simulink model "NMC_batt_model_80_1dot5C"  (R2023b)
settings: Solver=FixedStepAuto  StartTime=0.0  StopTime=10^7  FixedStep=50
undefined symbols (not defined in the file): DiscIntNeverNeededParam, sigbuilder_block
libraries: batteryecm_lib x100, fl_lib x15, nesl_utility x10, simulink x4, dspswit3 x2
(part 2 of 4)

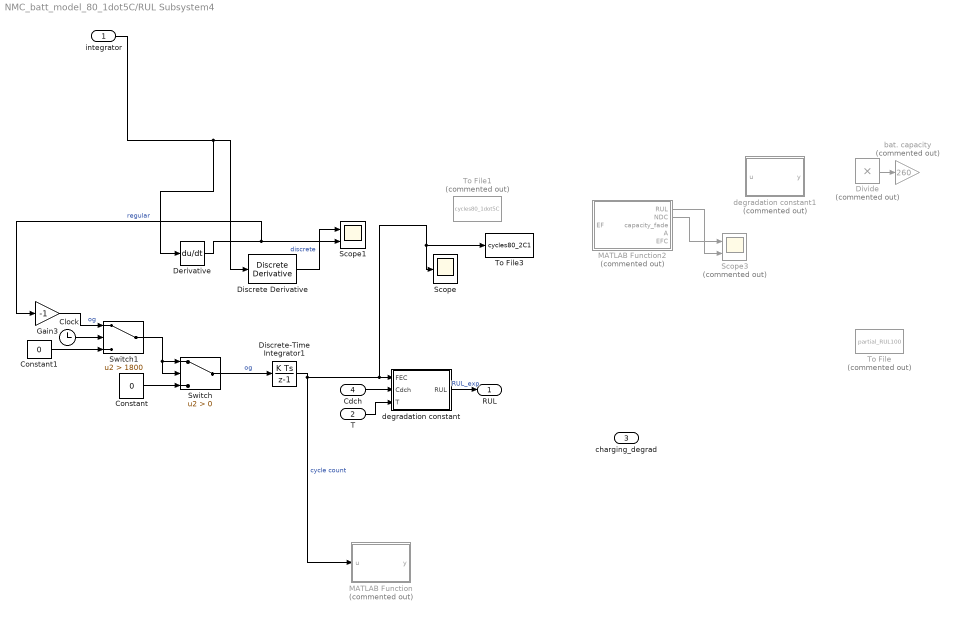
== system NMC_batt_model_80_1dot5C/RUL Subsystem4 ==
  integrator : Inport
  T : Inport  Port=2
  charging_degrad : Inport  Port=3
  Cdch : Inport  Port=4
  Clock : Clock
  Constant : Constant  Value=0
  Constant1 : Constant  Value=0
  Derivative : Derivative  CoefficientInTFapproximation=1000
  Discrete Derivative : simulink/Discrete/Discrete Derivative  gainval=1.0  ICPrevScaledInput=0.0  OutMin=[]  OutMax=[]  OutDataType=fixdt(1, 16)  OutScaling=2^-10  DoSatur=off
  Discrete-Time Integrator1 : DiscreteIntegrator  SampleTime=-1  ICPrevOutput=DiscIntNeverNeededParam  ICPrevScaledInput=DiscIntNeverNeededParam
  Divide : Product  Commented=on  Inputs=**
  Gain3 : Gain  Gain=-1
  MATLAB Function : MATLAB Function  Commented=on  TreatAsAtomicUnit=on
  MATLAB Function2 : MATLAB Function  Commented=on  TreatAsAtomicUnit=on
  Scope : Scope
  Scope1 : Scope  NumInputPorts=2
  Scope3 : Scope  Commented=on  NumInputPorts=2
  Switch : Switch  Criteria=u2 > Threshold  ZeroCross=off  SaturateOnIntegerOverflow=off  InputSameDT=off
  Switch1 : Switch  Criteria=u2 > Threshold  Threshold=1800  SaturateOnIntegerOverflow=off  InputSameDT=off
  To File : ToFile  Commented=on  Filename=partial_RUL100  SaveFormat=Timeseries
  To File1 : ToFile  Commented=on  Filename=cycles80_1dot5C  SaveFormat=Timeseries
  To File3 : ToFile  Filename=cycles80_2C1  SaveFormat=Timeseries
  bat. capacity : Gain  Commented=on  Gain=260
  degradation constant : MATLAB Function  TreatAsAtomicUnit=on
  degradation constant1 : MATLAB Function  Commented=on  TreatAsAtomicUnit=on
  RUL : Outport
  wires:
  Gain3/1 -> Switch1/1  "og"
  Constant/1 -> Switch/3
  Derivative/1 -> Gain3/1, Scope1/2  "regular"
  Discrete Derivative/1 -> Scope1/1  "discrete"
  Switch/1 -> Discrete-Time Integrator1/1  "og"
  integrator/1 -> Derivative/1, Discrete Derivative/1
  Discrete-Time Integrator1/1 -> MATLAB Function/1(u), To File3/1, Scope/1, degradation constant/1(FEC)  "cycle count"
  Clock/1 -> Switch1/2
  Constant1/1 -> Switch1/3
  Switch1/1 -> Switch/1, Switch/2
  Divide/1 -> bat. capacity/1
  MATLAB Function2/1(RUL) -> Scope3/2
  MATLAB Function2/2(NDC) -> Scope3/1
  Cdch/1 -> degradation constant/2(Cdch)
  T/1 -> degradation constant/3(T)
  degradation constant/1(RUL) -> RUL/1  "RUL_exp"

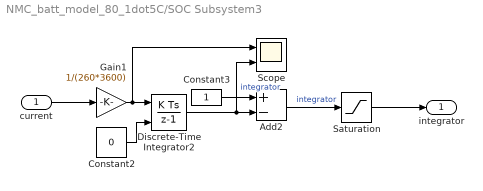
== system NMC_batt_model_80_1dot5C/SOC Subsystem3 ==
  current : Inport
  Add2 : Sum  Inputs=+-
  Constant2 : Constant  Value=0
  Constant3 : Constant
  Discrete-Time Integrator2 : DiscreteIntegrator  InitialConditionSource=external  SampleTime=-1  ICPrevOutput=DiscIntNeverNeededParam  ICPrevScaledInput=DiscIntNeverNeededParam
  Gain1 : Gain  Gain=1/(260*3600)
  Saturation : Saturate  UpperLimit=1  LowerLimit=0
  Scope : Scope  NumInputPorts=2
  integrator : Outport
  wires:
  Constant2/1 -> Discrete-Time Integrator2/2
  Constant3/1 -> Add2/1
  current/1 -> Gain1/1
  Gain1/1 -> Scope/1, Discrete-Time Integrator2/1
  Discrete-Time Integrator2/1 -> Scope/2, Add2/2  "integrator"
  Add2/1 -> Saturation/1  "integrator"
  Saturation/1 -> integrator/1

== system NMC_batt_model_80_1dot5C/Signal Builder ==
  Demux : Demux  Tag=STV Demux  Outputs=2
      settings: DisplayOption=none
  FromWs : FromWorkspace  Tag=STV FromWs  VariableName=tuvar
      SigBuilderData=|
      | common.afterFinalStr = 'Extrapolate'
      | common.sampleTime = 0
      | dataSet.timeRange = [0 2300]
      | dataSet.name = 'Group 1'
      | sbobj.Groups.Name = 'Group 1'
      | sbobj.Groups.Signals(1).Name = 'Signal 1'
      | sbobj.Groups.Signals(1).XData = [0 240 240 400 400 550 550 1600 1620 1650 1650 2300]
      | sbobj.Groups.Signals(1).YData = [30 31.5 40 40 38 38 36 36 33 33 0 0]
      | sbobj.Groups.Signals(2).Name = 'Signal 2'
      | sbobj.Groups.Signals(2).XData = [0 920 920 1380 1380 2300]
      | sbobj.Groups.Signals(2).YData = [0 0.045 1 1 0 0]
      | sbobj.Groups.TimeRange = [0 2300]
  Signal 1 : Outport  Tag=STV Outport
  Signal 2 : Outport  Tag=STV Outport  Port=2
  wires:
  Demux/1 -> Signal 1/1
  FromWs/1 -> Demux/1
  Demux/2 -> Signal 2/1

== system NMC_batt_model_80_1dot5C/Signal Builder1 ==
  Demux : Demux  Tag=STV Demux  Outputs=1
      settings: DisplayOption=none
  FromWs : FromWorkspace  Tag=STV FromWs  VariableName=tuvar
      SigBuilderData=|
      | common.afterFinalStr = 'Extrapolate'
      | common.sampleTime = 0
      | dataSet.timeRange = [0 4950]
      | dataSet.name = 'Group 1'
      | sbobj.Groups.Name = 'Group 1'
      | sbobj.Groups.Signals(1).Name = 'Signal 1'
      | sbobj.Groups.Signals(1).XData = [0 433 447 487 493 505 510 510 516 522 528 534 540 546 552 564 570 576 606 612 618 624 631 638 644 650 657 724 736 1176 1182 4661 4667 4711 4731 4743 4749 4755 4761 4767 4773 4785 4791 4835 4841 4847 4859 4865 4871 4877 4883 4889 4895 4927 4950]
      | sbobj.Groups.Signals(1).YData = [31.3 31.3 30.01 29.95 30.4 34.18 35.11 35.08 35.13 35.25 32.68 35.08 34 29.22 30.45 30.45 31.8 30.54 30.44 31.87 32.15 31.7 32.04 32.05 31.05 37.653 39.94 39.78 39.213 39.173 38.95 38.83 37.77 34.38 33.85 36.64 36.64 36.31 32.45 30.92 30.22 29.84 29.29 29.29 33.45 33.52 30.72 30.44 30.57 31 30.92 30.97 30.08 30 30]
      | sbobj.Groups.Signals(2).Name = 'Signal 2'
      | sbobj.Groups.Signals(2).XData = [0 920 920 1380 1380 2300]
      | sbobj.Groups.Signals(2).YData = [0 0.045 1 1 0 0]
      | sbobj.Groups.TimeRange = [0 4950]
  Signal 1 : Outport  Tag=STV Outport
  wires:
  Demux/1 -> Signal 1/1
  FromWs/1 -> Demux/1

== system NMC_batt_model_80_1dot5C/Signal Builder3 ==
  Demux : Demux  Tag=STV Demux  Outputs=1
      settings: DisplayOption=none
  FromWs : FromWorkspace  Tag=STV FromWs  VariableName=tuvar
      SigBuilderData=|
      | common.afterFinalStr = 'Extrapolate'
      | common.sampleTime = 0
      | dataSet.timeRange = [0 1800]
      | dataSet.name = 'Group 1'
      | sbobj.Groups.Name = 'Group 1'
      | sbobj.Groups.Signals(1).Name = 'Signal 1'
      | sbobj.Groups.Signals(1).XData = [0 150 155 160 170 175 175 228 230 240 936 936 1680 1700 1720 1790 1790 2300]
      | sbobj.Groups.Signals(1).YData = [30 30 33.5 34 33.5 30 29 30.5 30.1 38.5 38.5 36 36 33 30.5 30 0 0]
      | sbobj.Groups.Signals(2).Name = 'Signal 2'
      | sbobj.Groups.Signals(2).XData = [0 920 920 1380 1380 2300]
      | sbobj.Groups.Signals(2).YData = [0 0.045 1 1 0 0]
      | sbobj.Groups.TimeRange = [0 2300]
  Signal 1 : Outport  Tag=STV Outport
  wires:
  Demux/1 -> Signal 1/1
  FromWs/1 -> Demux/1

== system NMC_batt_model_80_1dot5C/Subsystem ==
  Subsystem : Subsystem
  Subsystem1 : Subsystem
  Subsystem2 : Subsystem
  Subsystem3 : Subsystem
  + : PMIOPort  Side=Left
  - : PMIOPort  Port=2  Side=Right
  SOC : Outport
  wires:
  Subsystem/1(SOC) -> SOC/1
  connections:
  +/RConn1 -- Subsystem/LConn1
  Subsystem1/LConn1 -- Subsystem/RConn1
  Subsystem2/LConn1 -- Subsystem1/RConn1
  Subsystem3/LConn1 -- Subsystem2/RConn1
  -/RConn1 -- Subsystem3/RConn1

== system NMC_batt_model_80_1dot5C/Subsystem1 ==
  SOC : Inport
  MATLAB Function : MATLAB Function  TreatAsAtomicUnit=on
  Unit Delay : UnitDelay  SampleTime=-1  HasFrameUpgradeWarning=on
  y : Outport
  wires:
  MATLAB Function/1(y) -> Unit Delay/1, y/1
  SOC/1 -> MATLAB Function/2(SOC)
  Unit Delay/1 -> MATLAB Function/1("y ")

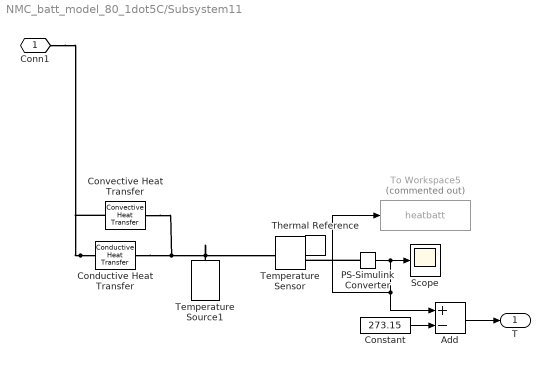
== system NMC_batt_model_80_1dot5C/Subsystem11 ==
  Add : Sum  Inputs=+-
  Conductive Heat Transfer : fl_lib/Thermal/Thermal Elements/Conductive Heat Transfer  thermal_type=foundation.enum.ConstantVariableTabulated.Constant  wall_geometry=foundation.enum.ConductionWallGeometry.Planar  area=1e-4 m^2  thickness=0.1 m  d_in=0.05 m  d_out=0.1 m  L=1 m  th_cond_min=10 W/(K*m)  th_cond=401 W/(K*m)  th_cond_TLU=[413, 401, 392, 383, 371, 357, 342] W/(K*m)  temp_TLU=[200, 273, 400, 600, 800, 1000, 1200] K  T_specify=off  T_priority=None  T=0 K  T_nominal_specify=off  T_nominal_unit=K  T_nominal_value=1  Q_specify=off  Q_priority=None  Q=0 W  Q_nominal_specify=off  Q_nominal_unit=W  Q_nominal_value=1
  Constant : Constant  Value=273.15
  Convective Heat Transfer : fl_lib/Thermal/Thermal Elements/Convective Heat Transfer  thermal_type=foundation.enum.constant_variable.constant  area=1e-4 m^2  heat_tr_coeff=20 W/(K*m^2)  min_heat_tr_coeff=1e-3 W/(K*m^2)  T_specify=off  T_priority=None  T=0 K  T_nominal_specify=off  T_nominal_unit=K  T_nominal_value=1  Q_specify=off  Q_priority=None  Q=0 W  Q_nominal_specify=off  Q_nominal_unit=W  Q_nominal_value=1
  PS-Simulink Converter : nesl_utility/PS-Simulink Converter  PhysicalDomain=network_engine_domain  SubClassName=ps_output  LeftPortType=input  RightPortType=output  PseudoPeriodic=off  Frequencies=[]  VectorFormat=inherit  Unit=inherit  AffineConversion=off
  Scope : Scope
  Temperature Sensor : fl_lib/Thermal/Thermal Sensors/Temperature Sensor  temperature_measure=foundation.enum.MeasurementReference.difference
  Temperature Source1 : fl_lib/Thermal/Thermal Sources/Temperature Source  temperature=293.15 K
  Thermal Reference : fl_lib/Thermal/Thermal Elements/Thermal Reference
  To Workspace5 : ToWorkspace  Commented=on  VariableName=heatbatt  SaveFormat=Structure With Time  SampleTime=-1
      settings: Decimation=1000
  Conn1 : PMIOPort  Side=Left
  T : Outport
  wires:
  PS-Simulink Converter/1 -> Add/1, To Workspace5/1, Scope/1
  Add/1 -> T/1
  Constant/1 -> Add/2
  connections:
  Thermal Reference/LConn1 -- Temperature Sensor/RConn1
  Conductive Heat Transfer/RConn1 -- Convective Heat Transfer/RConn1 -- Temperature Source1/LConn1 -- Temperature Sensor/LConn1
  Conductive Heat Transfer/LConn1 -- Conn1/RConn1 -- Convective Heat Transfer/LConn1
  PS-Simulink Converter/LConn1 -- Temperature Sensor/RConn2

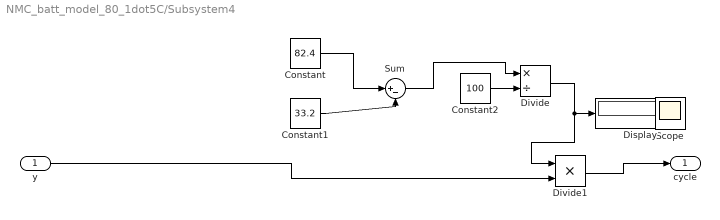
== system NMC_batt_model_80_1dot5C/Subsystem4 ==
  y : Inport
  Constant : Constant  Value=82.4
  Constant1 : Constant  Value=33.2
  Constant2 : Constant  Value=100
  Display : Display
  Divide : Product  Inputs=*/
  Divide1 : Product  Inputs=**
  Scope : Scope
  Sum : Sum  Inputs=|+-
  cycle : Outport
  wires:
  Constant/1 -> Sum/1
  Constant1/1 -> Sum/2
  Divide/1 -> Divide1/1, Display/1
  y/1 -> Divide1/2
  Divide1/1 -> cycle/1
  Constant2/1 -> Divide/2
  Sum/1 -> Divide/1

== system NMC_batt_model_80_1dot5C/charge regulation1 ==
  subSOC : Inport
  sig : Inport  Port=2
  Clock : Clock
  MATLAB Function2 : MATLAB Function  TreatAsAtomicUnit=on
  Unit Delay : UnitDelay  InitialCondition=-1  SampleTime=-1  HasFrameUpgradeWarning=on
  y : Outport
  wires:
  MATLAB Function2/1(y) -> Unit Delay/1, y/1
  Unit Delay/1 -> MATLAB Function2/1("y ")
  Clock/1 -> MATLAB Function2/2(t)
  subSOC/1 -> MATLAB Function2/3(SOC)
  sig/1 -> MATLAB Function2/4(sig)

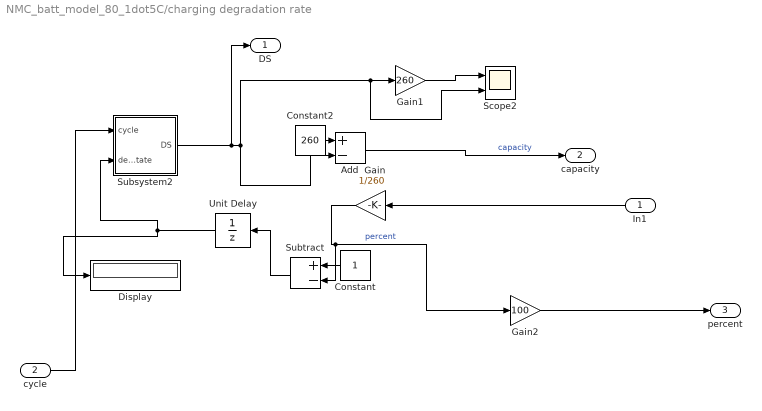
== system NMC_batt_model_80_1dot5C/charging degradation rate ==
  In1 : Inport
  cycle : Inport  Port=2
  Add : Sum  Inputs=+-
  Constant : Constant
  Constant2 : Constant  Value=260
  Display : Display
  Gain : Gain  Gain=1/260
  Gain1 : Gain  Gain=260
  Gain2 : Gain  Gain=100
  Scope2 : Scope  NumInputPorts=2
  Subsystem2 : Subsystem
  Subtract : Sum  Inputs=+-
  Unit Delay : UnitDelay  SampleTime=-1  HasFrameUpgradeWarning=on
  DS : Outport
  capacity : Outport  Port=2
  percent : Outport  Port=3
  wires:
  Unit Delay/1 -> Subsystem2/2(degradation_state), Display/1
  Subsystem2/1(DS) -> DS/1, Add/2, Scope2/2, Gain1/1
  cycle/1 -> Subsystem2/1(cycle)
  Constant2/1 -> Add/1
  Gain/1 -> Gain2/1, Subtract/2  "percent"
  Add/1 -> capacity/1  "capacity"
  In1/1 -> Gain/1
  Gain1/1 -> Scope2/1
  Constant/1 -> Subtract/1
  Subtract/1 -> Unit Delay/1
  Gain2/1 -> percent/1

== system NMC_batt_model_80_1dot5C/cycle counter ==
  subSOC : Inport
  Compare To Constant : simulink/Logic and Bit Operations/Compare To Constant  relop=>=  const=0.8  OutDataTypeStr=boolean
  Counter : dspswit3/Counter  Direction=Up  CountEvent=Rising edge  CounterSize=User defined  MaxCount=10000  InitialCount=0  Output=Count and Hit  HitValue=32  ResetInput=off  SamplesPerFrame=1  Ts=1  CntDtype=double  HitDtype=Logical
  Edge Detector1 : dspswit3/Edge Detector  InputProcessing=Columns as channels (frame based)
  Scope31 : Scope  NumInputPorts=2
  cnt : Outport
  hit : Outport  Port=2
  wires:
  Counter/1 -> cnt/1  "cnt"
  Compare To Constant/1 -> Edge Detector1/1, Scope31/1
  Edge Detector1/1 -> Counter/1, Scope31/2  "edge"
  subSOC/1 -> Compare To Constant/1
  Counter/2 -> hit/1  "hit"

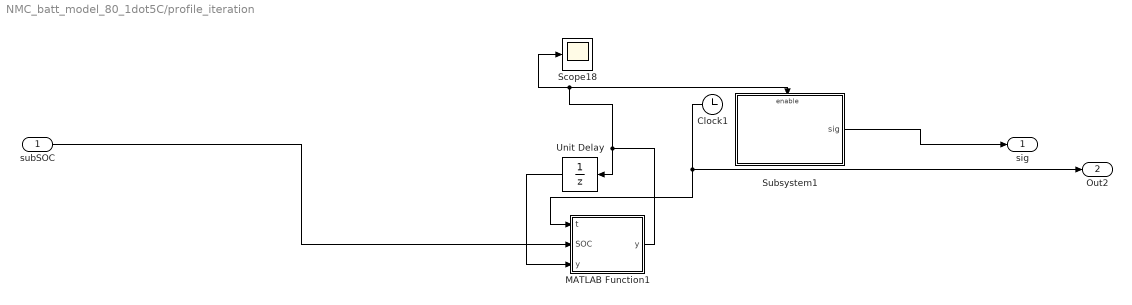
== system NMC_batt_model_80_1dot5C/profile_iteration ==
  subSOC : Inport
  Clock1 : Clock
  MATLAB Function1 : MATLAB Function  TreatAsAtomicUnit=on
  Scope18 : Scope
  Subsystem1 : Subsystem
  Unit Delay : UnitDelay  SampleTime=-1  HasFrameUpgradeWarning=on
  sig : Outport
  Out2 : Outport  Port=2
  wires:
  Subsystem1/1(sig) -> sig/1
  Clock1/1 -> Out2/1, MATLAB Function1/1(t)
  MATLAB Function1/1(y) -> Scope18/1, Subsystem1/Enable, Unit Delay/1
  Unit Delay/1 -> MATLAB Function1/3("y ")
  subSOC/1 -> MATLAB Function1/2(SOC)

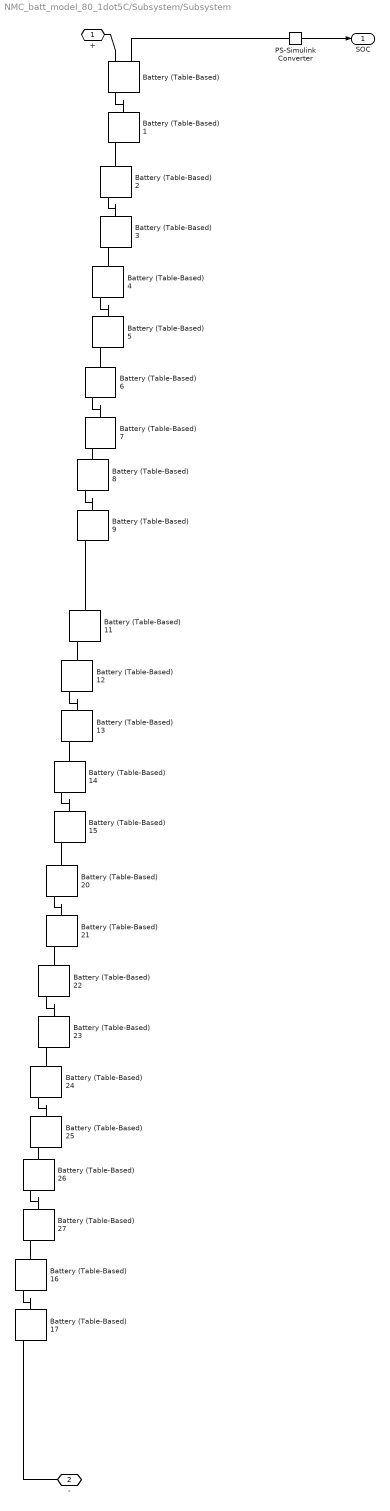
== system NMC_batt_model_80_1dot5C/Subsystem/Subsystem ==
  Battery (Table-Based) : batteryecm_lib/Battery (Table-Based)  Tag={'toolbox/physmod/battery/shared_library/m/batteryecm_lib_parts';'Battery__Table_Based_/Panasonic/NCR18650PF.xml'}  SOC_vec=[0 0.01 0.02 0.03 0.04 0.05 0.06 0.07 0.08 0.09 0.1 0.11 0.12 0.13 0.14 0.15 0.16 0.17 0.18 0.19 0.2 0.21 0.22 0.23 0.24 0.25 0.26 0.27 0.28 0.29 0.3 0.31 0.32 0.33 0.34 0.35 0.36 0.37 0.38 0.39 0.4 0.41 0.42 0.43 0.44 0.45 0.46 0.47 0.48 0.49 0.5 0.51 0.52 0.53 0.54 0.55 0.56 0.57 0.58 0.59 0.6 0.61 0.62 0.63 0.64 0.65 0.66 0.67 0.68 0.69 0.7 0.71 0.72 0.73 0.74 0.75 0.76 0.77 0.78 0.79 0.8 0.81 0.82 0.83 0.84 0.85 0.86 0.87 0.88 0.89 0.9 0.91 0.92 0.93 0.94 0.95 0.96 0.97 0.98 0.99 1]  T_dependence=simscape.enum.tablebattery.temperature_dependence.yes  prm_dir=simscape.enum.tablebattery.prm_dir.noCurrentDirectionality  T_vec=[-10 0 25 45] degC  V0_mat=[2.80555 2.80555 2.80555 2.80555;2.85959 2.85959 2.85959 2.85959;2.91363 2.91363 2.91363 2.91363;3.00304 3.00304 3.00304 3.00304;3.0606 3.0606 3.0606 3.0606;3.09933 3.09933 3.09933 3.09933;3.12978 3.12978 3.12978 3.12978;3.18381 3.18381 3.18381 3.18381;3.23096 3.23096 3.23096 3.23096;3.26469 3.26469 3.26469 3.26469;3.2911 3.2911 3.2911 3.2911;3.31202 3.31202 3.31202 3.31202;3.33368 3.33368 3.33368 3.33368;3.35023 3.35023 3.35023 3.35023;3.3665 3.3665 3.3665 3.3665;3.38187 3.38187 3.38187 3.38187;3.39652 3.39652 3.39652 3.39652;3.40935 3.40935 3.40935 3.40935;3.42296 3.42296 3.42296 3.42296;3.43602 3.43602 3.43602 3.43602;3.4475 3.4475 3.4475 3.4475;3.45894 3.45894 3.45894 3.45894;3.46943 3.46943 3.46943 3.46943;3.47583 3.47583 3.47583 3.47583;3.48131 3.48131 3.48131 3.48131;3.48929 3.48929 3.48929 3.48929;3.49863 3.49863 3.49863 3.49863;3.50723 3.50723 3.50723 3.50723;3.51419 3.51419 3.51419 3.51419;3.52064 3.52064 3.52064 3.52064;3.52703 3.52703 3.52703 3.52703;3.53288 3.53288 3.53288 3.53288;3.5383 3.5383 3.5383 3.5383;3.54248 3.54248 3.54248 3.54248;3.54635 3.54635 3.54635 3.54635;3.55067 3.55067 3.55067 3.55067;3.55538 3.55538 3.55538 3.55538;3.56162 3.56162 3.56162 3.56162;3.56772 3.56772 3.56772 3.56772;3.57355 3.57355 3.57355 3.57355;3.57907 3.57907 3.57907 3.57907;3.58466 3.58466 3.58466 3.58466;3.59099 3.59099 3.59099 3.59099;3.59795 3.59795 3.59795 3.59795;3.60491 3.60491 3.60491 3.60491;3.61176 3.61176 3.61176 3.61176;3.61856 3.61856 3.61856 3.61856;3.62438 3.62438 3.62438 3.62438;3.62996 3.62996 3.62996 3.62996;3.63625 3.63625 3.63625 3.63625;3.64309 3.64309 3.64309 3.64309;3.64978 3.64978 3.64978 3.64978;3.65633 3.65633 3.65633 3.65633;3.66344 3.66344 3.66344 3.66344;3.67149 3.67149 3.67149 3.67149;3.67995 3.67995 3.67995 3.67995;3.68883 3.68883 3.68883 3.68883;3.69977 3.69977 3.69977 3.69977;3.7106 3.7106 3.7106 3.7106;3.72128 3.72128 3.72128 3.72128;3.72977 3.72977 3.72977 3.72977;3.73862 3.73862 3.73862 3.73862;3.74839 3.74839 3.74839 3.74839;3.75854 3.75854 3.75854 3.75854;3.76808 3.76808 3.76808 3.76808;3.77731 3.77731 3.77731 3.77731;3.78691 3.78691 3.78691 3.78691;3.79724 3.79724 3.79724 3.79724;3.80748 3.80748 3.80748 3.80748;3.817 3.817 3.817 3.817;3.82465 3.82465 3.82465 3.82465;3.83227 3.83227 3.83227 3.83227;3.8402 3.8402 3.8402 3.8402;3.84937 3.84937 3.84937 3.84937;3.85948 3.85948 3.85948 3.85948;3.87001 3.87001 3.87001 3.87001;3.88001 3.88001 3.88001 3.88001;3.88909 3.88909 3.88909 3.88909;3.89708 3.89708 3.89708 3.89708;3.90554 3.90554 3.90554 3.90554;3.91623 3.91623 3.91623 3.91623;3.9276 3.9276 3.9276 3.9276;3.9408 3.9408 3.9408 3.9408;3.95458 3.95458 3.95458 3.95458;3.96671 3.96671 3.96671 3.96671;3.97597 3.97597 3.97597 3.97597;3.98588 3.98588 3.98588 3.98588;3.99921 3.99921 3.99921 3.99921;4.01279 4.01279 4.01279 4.01279;4.02654 4.02654 4.02654 4.02654;4.03959 4.03959 4.03959 4.03959;4.05214 4.05214 4.05214 4.05214;4.06294 4.06294 4.06294 4.06294;4.07257 4.07257 4.07257 4.07257;4.08033 4.08033 4.08033 4.08033;4.08863 4.08863 4.08863 4.08863;4.09953 4.09953 4.09953 4.09953;4.11328 4.11328 4.11328 4.11328;4.13091 4.13091 4.13091 4.13091;4.15201 4.15201 4.15201 4.15201;4.17387 4.17387 4.17387 4.17387] V  V0_vec=[2.80555 2.85959 2.91363 3.00304 3.0606 3.09933 3.12978 3.18381 3.23096 3.26469 3.2911 3.31202 3.33368 3.35023 3.3665 3.38187 3.39652 3.40935 3.42296 3.43602 3.4475 3.45894 3.46943 3.47583 3.48131 3.48929 3.49863 3.50723 3.51419 3.52064 3.52703 3.53288 3.5383 3.54248 3.54635 3.55067 3.55538 3.56162 3.56772 3.57355 3.57907 3.58466 3.59099 3.59795 3.60491 3.61176 3.61856 3.62438 3.62996 3.63625 3.64309 3.64978 3.65633 3.66344 3.67149 3.67995 3.68883 3.69977 3.7106 3.72128 3.72977 3.73862 3.74839 3.75854 3.76808 3.77731 3.78691 3.79724 3.80748 3.817 3.82465 3.83227 3.8402 3.84937 3.85948 3.87001 3.88001 3.88909 3.89708 3.90554 3.91623 3.9276 3.9408 3.95458 3.96671 3.97597 3.98588 3.99921 4.01279 4.02654 4.03959 4.05214 4.06294 4.07257 4.08033 4.08863 4.09953 4.11328 4.13091 4.15201 4.17387] V  V_range=[2.25 Inf] V  R0_mat=[0.75549 0.67245 0.17403 0.112;0.85269 0.75703 0.14702 0.03414;0.81792 0.71964 0.12022 0.00255;0.78315 0.68225 0.10415 2e-05;0.74837 0.64486 0.08835 2e-05;0.7136 0.60747 0.07462 2e-05;0.67883 0.57008 0.06392 2e-05;0.64406 0.53269 0.06243 0.01154;0.60929 0.49529 0.06276 0.02196;0.57452 0.4579 0.06157 0.02895;0.53975 0.42051 0.06015 0.03291;0.50498 0.38312 0.0587 0.03446;0.47021 0.34573 0.05791 0.03749;0.43544 0.30834 0.05742 0.03912;0.40067 0.27163 0.05726 0.04077;0.3659 0.2399 0.05695 0.04312;0.33113 0.21598 0.05669 0.04519;0.29855 0.19556 0.0563 0.04597;0.27187 0.18199 0.05643 0.04689;0.25149 0.16998 0.05637 0.04778;0.23672 0.15947 0.05613 0.04881;0.22094 0.15288 0.05627 0.04983;0.21055 0.14641 0.0562 0.05042;0.19955 0.13998 0.0555 0.04905;0.19137 0.13379 0.05463 0.04734;0.18464 0.13036 0.05424 0.0468;0.17901 0.12743 0.05396 0.04733;0.17336 0.12471 0.05353 0.04759;0.16963 0.12142 0.05325 0.04697;0.16579 0.11998 0.053 0.04616;0.16242 0.11856 0.05273 0.04563;0.15887 0.11696 0.05239 0.04515;0.15558 0.1153 0.05185 0.04523;0.15182 0.11319 0.05104 0.04515;0.14868 0.11098 0.05016 0.04495;0.14619 0.10898 0.0496 0.04427;0.1438 0.10712 0.04917 0.0435;0.14196 0.10583 0.049 0.0433;0.14006 0.10467 0.04873 0.04342;0.13885 0.1036 0.04841 0.04343;0.13751 0.10241 0.04805 0.04333;0.13605 0.10125 0.04775 0.04289;0.13479 0.10081 0.04765 0.04219;0.13386 0.10079 0.04766 0.04172;0.13314 0.10076 0.04767 0.04125;0.13237 0.10071 0.04767 0.04141;0.13163 0.10106 0.04767 0.04164;0.13057 0.10103 0.04746 0.04127;0.12942 0.10092 0.04718 0.04039;0.12835 0.0993 0.04683 0.03977;0.12742 0.09756 0.04661 0.03935;0.12651 0.09576 0.04638 0.03877;0.12576 0.09551 0.04611 0.03814;0.12522 0.09549 0.04546 0.03775;0.12534 0.0958 0.04498 0.03789;0.12567 0.09566 0.0446 0.03806;0.12544 0.09568 0.04436 0.03754;0.12563 0.09645 0.0447 0.03778;0.12579 0.09742 0.0452 0.03809;0.12561 0.09838 0.04568 0.03858;0.12463 0.09848 0.04568 0.03827;0.12444 0.09858 0.04565 0.03791;0.12488 0.09902 0.04553 0.03774;0.12541 0.0989 0.04551 0.03771;0.12553 0.09832 0.04545 0.0378;0.12554 0.09763 0.04533 0.03827;0.12569 0.09779 0.04532 0.03888;0.12679 0.09822 0.0455 0.03964;0.12813 0.09884 0.04565 0.03957;0.12921 0.09949 0.04568 0.03924;0.12875 0.09944 0.04547 0.03856;0.12761 0.09947 0.04525 0.03793;0.12678 0.09962 0.04509 0.0374;0.12741 0.10014 0.04486 0.03728;0.12819 0.10071 0.04471 0.03749;0.12866 0.10143 0.04473 0.03825;0.12934 0.10218 0.04488 0.0389;0.13071 0.10266 0.04509 0.03921;0.13167 0.10268 0.04508 0.03827;0.13235 0.10275 0.04519 0.03748;0.13367 0.10365 0.04567 0.03751;0.13524 0.10475 0.0459 0.03791;0.1378 0.10652 0.04653 0.03898;0.14098 0.10898 0.04736 0.0402;0.14355 0.11127 0.04774 0.04039;0.14492 0.11249 0.04743 0.03953;0.1465 0.11343 0.04723 0.03861;0.14934 0.11546 0.04771 0.03891;0.15255 0.11759 0.04823 0.0391;0.15585 0.12007 0.04878 0.03936;0.15888 0.12238 0.04933 0.0398;0.16256 0.12454 0.04973 0.04018;0.16629 0.12609 0.0497 0.03988;0.16958 0.1272 0.04945 0.03914;0.1737 0.12779 0.0488 0.0377;0.17938 0.12952 0.04782 0.03647;0.18591 0.1322 0.04663 0.0362;0.19342 0.13509 0.04586 0.03591;0.20235 0.13879 0.04557 0.03672;0.20886 0.14194 0.04146 0.03487;0.20094 0.13122 0.03511 0.0299] Ohm  R0_vec=[0.17403 0.14702 0.12022 0.10415 0.08835 0.07462 0.06392 0.06243 0.06276 0.06157 0.06015 0.0587 0.05791 0.05742 0.05726 0.05695 0.05669 0.0563 0.05643 0.05637 0.05613 0.05627 0.0562 0.0555 0.05463 0.05424 0.05396 0.05353 0.05325 0.053 0.05273 0.05239 0.05185 0.05104 0.05016 0.0496 0.04917 0.049 0.04873 0.04841 0.04805 0.04775 0.04765 0.04766 0.04767 0.04767 0.04767 0.04746 0.04718 0.04683 0.04661 0.04638 0.04611 0.04546 0.04498 0.0446 0.04436 0.0447 0.0452 0.04568 0.04568 0.04565 0.04553 0.04551 0.04545 0.04533 0.04532 0.0455 0.04565 0.04568 0.04547 0.04525 0.04509 0.04486 0.04471 0.04473 0.04488 0.04509 0.04508 0.04519 0.04567 0.0459 0.04653 0.04736 0.04774 0.04743 0.04723 0.04771 0.04823 0.04878 0.04933 0.04973 0.0497 0.04945 0.0488 0.04782 0.04663 0.04586 0.04557 0.04146 0.03511] Ohm  R0_dis_mat=[.0117, .0085, .009; .011, .0085, .009; .0114, .0087, .0092; .0107, .0082, .0088; .0107, .0083, .0091; .0113, .0085, .0089; .0116, .0085, .0089] % Parameter not set Ohm  R0_dis_vec=[.0085, .0085, .0087, .0082, .0083, .0085, .0085] % Parameter not set Ohm  R0_ch_mat=[.0117, .0085, .009; .011, .0085, .009; .0114, .0087, .0092; .0107, .0082, .0088; .0107, .0083, .0091; .0113, .0085, .0089; .0116, .0085, .0089] % Parameter not set Ohm  R0_ch_vec=[.0085, .0085, .0087, .0082, .0083, .0085, .0085] % Parameter not set Ohm  AH=260 hr*A  prm_leak=simscape.enum.tablebattery.prm_leak.disabled  Rleak_vec=[8000, 7000, 6000] % Parameter not set Ohm  Rleak=7e3 % Parameter not set Ohm  extrapolation_option=simscape.enum.extrapolation.nearest  SOC_port=simscape.enum.tablebattery.enable.yes  prm_dyn=simscape.enum.tablebattery.prm_dyn.off  R1_mat=[.0109, .0029, .0013; .0069, .0024, .0012; .0047, .0026, .0013; .0034, .0016, .001; .0033, .0023, .0014; .0033, .0018, .0011; .0028, .0017, .0011] % Parameter not set Ohm  R1_vec=[.0029, .0024, .0026, .0016, .0023, .0018, .0017] % Parameter not set Ohm  tau1_mat=[20, 36, 39; 31, 45, 39; 109, 105, 61; 36, 29, 26; 59, 77, 67; 40, 33, 29; 25, 39, 33] % Parameter not set s  tau1_vec=[36, 45, 105, 29, 77, 33, 39] % Parameter not set s  R2_mat=[.0109, .0029, .0013; .0069, .0024, .0012; .0047, .0026, .0013; .0034, .0016, .001; .0033, .0023, .0014; .0033, .0018, .0011; .0028, .0017, .0011] % Parameter not set Ohm  R2_vec=[.0029, .0024, .0026, .0016, .0023, .0018, .0017] % Parameter not set Ohm  tau2_mat=[20, 36, 39; 31, 45, 39; 109, 105, 61; 36, 29, 26; 59, 77, 67; 40, 33, 29; 25, 39, 33] % Parameter not set s  tau2_vec=[36, 45, 105, 29, 77, 33, 39] % Parameter not set s  R3_mat=[.0109, .0029, .0013; .0069, .0024, .0012; .0047, .0026, .0013; .0034, .0016, .001; .0033, .0023, .0014; .0033, .0018, .0011; .0028, .0017, .0011] % Parameter not set Ohm  R3_vec=[.0029, .0024, .0026, .0016, .0023, .0018, .0017] % Parameter not set Ohm  tau3_mat=[20, 36, 39; 31, 45, 39; 109, 105, 61; 36, 29, 26; 59, 77, 67; 40, 33, 29; 25, 39, 33] % Parameter not set s  tau3_vec=[36, 45, 105, 29, 77, 33, 39] % Parameter not set s  R4_mat=[.0109, .0029, .0013; .0069, .0024, .0012; .0047, .0026, .0013; .0034, .0016, .001; .0033, .0023, .0014; .0033, .0018, .0011; .0028, .0017, .0011] % Parameter not set Ohm  R4_vec=[.0029, .0024, .0026, .0016, .0023, .0018, .0017] % Parameter not set Ohm  tau4_mat=[20, 36, 39; 31, 45, 39; 109, 105, 61; 36, 29, 26; 59, 77, 67; 40, 33, 29; 25, 39, 33] % Parameter not set s  tau4_vec=[36, 45, 105, 29, 77, 33, 39] % Parameter not set s  R5_mat=[.0109, .0029, .0013; .0069, .0024, .0012; .0047, .0026, .0013; .0034, .0016, .001; .0033, .0023, .0014; .0033, .0018, .0011; .0028, .0017, .0011] % Parameter not set Ohm  R5_vec=[.0029, .0024, .0026, .0016, .0023, .0018, .0017] % Parameter not set Ohm  tau5_mat=[20, 36, 39; 31, 45, 39; 109, 105, 61; 36, 29, 26; 59, 77, 67; 40, 33, 29; 25, 39, 33] % Parameter not set s  tau5_vec=[36, 45, 105, 29, 77, 33, 39] % Parameter not set s  prm_fade=simscape.enum.tablebattery.prm_fade.tableN  N0=100 % Parameter not set  dV0=0 % Parameter not set  dR0=0 % Parameter not set  dAH=0 % Parameter not set  dRleak=0 % Parameter not set  dR1=0 % Parameter not set  dR2=0 % Parameter not set  dR3=0 % Parameter not set  dR4=0 % Parameter not set  dR5=0 % Parameter not set  N0vec=[0 7 13 19 25 31 37 43 49 55 61 67 73 79 85 91 97 103 109 115 121 127 133 139 145 151 157 163 169 175 181 187 193 199 205 211 217 223 229 235 241 247 253 259 265 271 277 283 289 295 301 307 313 319 325 331 337 343 349 355 361 367 373 379 385 391 397 403 409 415 421 427 433 439 445 451 457 463 469 475 481 487 493 499]  Tfadevec=[298.15, 323.15] % Parameter not set K  dV0vec=[0 -0.2132 -0.4265 -0.6357 -0.8415 -1.0444 -1.2163 -1.3883 -1.52 -1.6273 -1.7347 -1.8294 -1.9144 -1.9994 -2.0744 -2.1392 -2.204 -2.2607 -2.3098 -2.3589 -2.408 -2.4643 -2.5252 -2.5861 -2.647 -2.7238 -2.8051 -2.8864 -2.9759 -3.0704 -3.1649 -3.261 -3.3591 -3.4573 -3.5079 -3.5566 -3.6065 -3.6564 -3.7063 -3.7562 -3.8061 -3.8559 -3.9166 -3.9805 -4.0444 -4.1083 -4.1723 -4.2352 -4.2979 -4.3605 -4.4214 -4.4739 -4.5206 -4.5597 -4.5988 -4.6379 -4.6769 -4.716 -4.7547 -4.7957 -4.8368 -4.8778 -4.9188 -4.9598 -5.0123 -5.066 -5.1196 -5.1598 -5.1853 -5.2109 -5.2365 -5.2631 -5.2922 -5.3213 -5.3503 -5.3816 -5.4144 -5.4471 -5.4798 -5.5126 -5.5453 -5.578 -5.6097 -5.641]  dR0vec=[0 0 0 0 0 0 0 0 0 0 0 0 0 0 0 0 0 0 0 0 0 0 0 0 0 0 0 0 0 0 0 0 0 0 0 0 0 0 0 0 0 0 0 0 0 0 0 0 0 0 0 0 0 0 0 0 0 0 0 0 0 0 0 0 0 0 0 0 0 0 0 0 0 0 0 0 0 0 0 0 0 0 0 0] % Parameter assumed  dAHvec=[0 -0.407 -0.814 -1.221 -1.629 -2.036 -2.443 -2.85 -3.207 -3.533 -3.859 -4.185 -4.51 -4.836 -5.162 -5.488 -5.813 -6.105 -6.369 -6.633 -6.897 -7.161 -7.425 -7.689 -7.953 -8.255 -8.569 -8.883 -9.197 -9.511 -9.826 -10.14 -10.454 -10.768 -10.93 -11.081 -11.233 -11.384 -11.536 -11.687 -11.838 -11.99 -12.176 -12.372 -12.569 -12.765 -12.962 -13.158 -13.354 -13.551 -13.741 -13.906 -14.07 -14.235 -14.399 -14.564 -14.728 -14.893 -15.06 -15.244 -15.429 -15.614 -15.799 -15.983 -16.168 -16.353 -16.538 -16.676 -16.764 -16.852 -16.94 -17.028 -17.116 -17.204 -17.292 -17.387 -17.486 -17.585 -17.684 -17.783 -17.883 -17.982 -18.081 -18.18]  dRleakvec=[0, 0, 0] % Parameter not set  dR1vec=[0, 0, 0] % Parameter not set  dR2vec=[0, 0, 0] % Parameter not set  dR3vec=[0, 0, 0] % Parameter not set  dR4vec=[0, 0, 0] % Parameter not set  dR5vec=[0, 0, 0] % Parameter not set  dV0mat=[0, 0; 0, 0; 0, 0] % Parameter not set  dR0mat=[0, 0; 0, 0; 0, 0] % Parameter not set  dAHmat=[0, 0; 0, 0; 0, 0] % Parameter not set  dRleakmat=[0, 0; 0, 0; 0, 0] % Parameter not set  dR1mat=[0, 0; 0, 0; 0, 0] % Parameter not set  dR2mat=[0, 0; 0, 0; 0, 0] % Parameter not set  dR3mat=[0, 0; 0, 0; 0, 0] % Parameter not set  dR4mat=[0, 0; 0, 0; 0, 0] % Parameter not set  dR5mat=[0, 0; 0, 0; 0, 0] % Parameter not set  prm_age_modeling=simscape.enum.tablebattery.prm_age_modeling.equation  storage_dt_age_vec=[0] % Parameter not set d  storage_T_age_vec=[273] % Parameter not set K  prm_age_OCV=simscape.enum.tablebattery.prm_age_OCV.OCV  OCV_age=0.9 % Parameter not set  SOC_age=0.6 % Parameter not set  prm_age_resistance=simscape.enum.tablebattery.prm_age.disabled  OCV_scaling_age_resistance=2.2134e6 % Parameter not set  OCV_offset_age_resistance=1.632e6 % Parameter not set  temp_exp_age_resistance=0.515833569 % Parameter not set V  t_exp_age_resistance=0.75 % Parameter not set  T_age_vec_resistance=[273.15, 298.15, 323.15] % Parameter not set K  dt_age_vec_resistance=[90, 180, 270, 360] % Parameter not set d  dR0_age_vec=[0, 0, 0] % Parameter not set  t_meas_dR0_age=100 % Parameter not set d  dR0_age_mat=[0, 0, 0; 0, 0, 0; 0, 0, 0; 0, 0, 0] % Parameter not set  prm_age_capacity=simscape.enum.tablebattery.prm_age.disabled  OCV_scaling_age_capacity=1.5097e07 % Parameter not set  OCV_offset_age_capacity=8.3625e06 % Parameter not set  temp_exp_age_capacity=0.6011 % Parameter not set V  t_exp_age_capacity=0.75 % Parameter not set  T_age_vec_capacity=[273.15, 298.15, 323.15] % Parameter not set K  dt_age_vec_capacity=[90, 180, 270, 360] % Parameter not set d  dAH_age_vec=[0, 0, 0] % Parameter not set  t_meas_dAH_age=100 % Parameter not set d  dAH_age_mat=[0, 0, 0; 0, 0, 0; 0, 0, 0; 0, 0, 0] % Parameter not set  thermal_port=simscape.enum.thermaleffects.model  temperature=298.15 % Parameter not set K  thermal_mass=43.2 % Parameter assumed J/K  i_specify=off  i_priority=None  i=0 A  i_nominal_specify=off  i_nominal_unit=A  i_nominal_value=1  v_specify=off  v_priority=None  v=0 V  v_nominal_specify=off  v_nominal_unit=V  v_nominal_value=1  stateOfCharge_specify=off  stateOfCharge_priority=High  stateOfCharge=1  stateOfCharge_nominal_specify=off  stateOfCharge_nominal_unit=1  stateOfCharge_nominal_value=1  num_cycles_specify=off  num_cycles_priority=High  num_cycles=0  num_cycles_nominal_specify=off  num_cycles_nominal_unit=1  num_cycles_nominal_value=1  cell_temperature_specify=off  cell_temperature_priority=High  cell_temperature=298.15 K  cell_temperature_nominal_specify=off  cell_temperature_nominal_unit=K  cell_temperature_nominal_value=1
      settings: AttributesFormatString=Panasonic:NCR18650PF
      settings: LibrarySourceBlock=|
      | batt_lib/Cells/Battery
      | (Table-Based)
  Battery (Table-Based){1..9,11..17,20..27} (24 alike) : batteryecm_lib/Battery (Table-Based)  Tag={'toolbox/physmod/battery/shared_library/m/batteryecm_lib_parts';'Battery__Table_Based_/Panasonic/NCR18650PF.xml'}  SOC_vec=[0 0.01 0.02 0.03 0.04 0.05 0.06 0.07 0.08 0.09 0.1 0.11 0.12 0.13 0.14 0.15 0.16 0.17 0.18 0.19 0.2 0.21 0.22 0.23 0.24 0.25 0.26 0.27 0.28 0.29 0.3 0.31 0.32 0.33 0.34 0.35 0.36 0.37 0.38 0.39 0.4 0.41 0.42 0.43 0.44 0.45 0.46 0.47 0.48 0.49 0.5 0.51 0.52 0.53 0.54 0.55 0.56 0.57 0.58 0.59 0.6 0.61 0.62 0.63 0.64 0.65 0.66 0.67 0.68 0.69 0.7 0.71 0.72 0.73 0.74 0.75 0.76 0.77 0.78 0.79 0.8 0.81 0.82 0.83 0.84 0.85 0.86 0.87 0.88 0.89 0.9 0.91 0.92 0.93 0.94 0.95 0.96 0.97 0.98 0.99 1]  T_dependence=simscape.enum.tablebattery.temperature_dependence.yes  prm_dir=simscape.enum.tablebattery.prm_dir.noCurrentDirectionality  T_vec=[-10 0 25 45] degC  V0_mat=[2.80555 2.80555 2.80555 2.80555;2.85959 2.85959 2.85959 2.85959;2.91363 2.91363 2.91363 2.91363;3.00304 3.00304 3.00304 3.00304;3.0606 3.0606 3.0606 3.0606;3.09933 3.09933 3.09933 3.09933;3.12978 3.12978 3.12978 3.12978;3.18381 3.18381 3.18381 3.18381;3.23096 3.23096 3.23096 3.23096;3.26469 3.26469 3.26469 3.26469;3.2911 3.2911 3.2911 3.2911;3.31202 3.31202 3.31202 3.31202;3.33368 3.33368 3.33368 3.33368;3.35023 3.35023 3.35023 3.35023;3.3665 3.3665 3.3665 3.3665;3.38187 3.38187 3.38187 3.38187;3.39652 3.39652 3.39652 3.39652;3.40935 3.40935 3.40935 3.40935;3.42296 3.42296 3.42296 3.42296;3.43602 3.43602 3.43602 3.43602;3.4475 3.4475 3.4475 3.4475;3.45894 3.45894 3.45894 3.45894;3.46943 3.46943 3.46943 3.46943;3.47583 3.47583 3.47583 3.47583;3.48131 3.48131 3.48131 3.48131;3.48929 3.48929 3.48929 3.48929;3.49863 3.49863 3.49863 3.49863;3.50723 3.50723 3.50723 3.50723;3.51419 3.51419 3.51419 3.51419;3.52064 3.52064 3.52064 3.52064;3.52703 3.52703 3.52703 3.52703;3.53288 3.53288 3.53288 3.53288;3.5383 3.5383 3.5383 3.5383;3.54248 3.54248 3.54248 3.54248;3.54635 3.54635 3.54635 3.54635;3.55067 3.55067 3.55067 3.55067;3.55538 3.55538 3.55538 3.55538;3.56162 3.56162 3.56162 3.56162;3.56772 3.56772 3.56772 3.56772;3.57355 3.57355 3.57355 3.57355;3.57907 3.57907 3.57907 3.57907;3.58466 3.58466 3.58466 3.58466;3.59099 3.59099 3.59099 3.59099;3.59795 3.59795 3.59795 3.59795;3.60491 3.60491 3.60491 3.60491;3.61176 3.61176 3.61176 3.61176;3.61856 3.61856 3.61856 3.61856;3.62438 3.62438 3.62438 3.62438;3.62996 3.62996 3.62996 3.62996;3.63625 3.63625 3.63625 3.63625;3.64309 3.64309 3.64309 3.64309;3.64978 3.64978 3.64978 3.64978;3.65633 3.65633 3.65633 3.65633;3.66344 3.66344 3.66344 3.66344;3.67149 3.67149 3.67149 3.67149;3.67995 3.67995 3.67995 3.67995;3.68883 3.68883 3.68883 3.68883;3.69977 3.69977 3.69977 3.69977;3.7106 3.7106 3.7106 3.7106;3.72128 3.72128 3.72128 3.72128;3.72977 3.72977 3.72977 3.72977;3.73862 3.73862 3.73862 3.73862;3.74839 3.74839 3.74839 3.74839;3.75854 3.75854 3.75854 3.75854;3.76808 3.76808 3.76808 3.76808;3.77731 3.77731 3.77731 3.77731;3.78691 3.78691 3.78691 3.78691;3.79724 3.79724 3.79724 3.79724;3.80748 3.80748 3.80748 3.80748;3.817 3.817 3.817 3.817;3.82465 3.82465 3.82465 3.82465;3.83227 3.83227 3.83227 3.83227;3.8402 3.8402 3.8402 3.8402;3.84937 3.84937 3.84937 3.84937;3.85948 3.85948 3.85948 3.85948;3.87001 3.87001 3.87001 3.87001;3.88001 3.88001 3.88001 3.88001;3.88909 3.88909 3.88909 3.88909;3.89708 3.89708 3.89708 3.89708;3.90554 3.90554 3.90554 3.90554;3.91623 3.91623 3.91623 3.91623;3.9276 3.9276 3.9276 3.9276;3.9408 3.9408 3.9408 3.9408;3.95458 3.95458 3.95458 3.95458;3.96671 3.96671 3.96671 3.96671;3.97597 3.97597 3.97597 3.97597;3.98588 3.98588 3.98588 3.98588;3.99921 3.99921 3.99921 3.99921;4.01279 4.01279 4.01279 4.01279;4.02654 4.02654 4.02654 4.02654;4.03959 4.03959 4.03959 4.03959;4.05214 4.05214 4.05214 4.05214;4.06294 4.06294 4.06294 4.06294;4.07257 4.07257 4.07257 4.07257;4.08033 4.08033 4.08033 4.08033;4.08863 4.08863 4.08863 4.08863;4.09953 4.09953 4.09953 4.09953;4.11328 4.11328 4.11328 4.11328;4.13091 4.13091 4.13091 4.13091;4.15201 4.15201 4.15201 4.15201;4.17387 4.17387 4.17387 4.17387] V  V0_vec=[2.80555 2.85959 2.91363 3.00304 3.0606 3.09933 3.12978 3.18381 3.23096 3.26469 3.2911 3.31202 3.33368 3.35023 3.3665 3.38187 3.39652 3.40935 3.42296 3.43602 3.4475 3.45894 3.46943 3.47583 3.48131 3.48929 3.49863 3.50723 3.51419 3.52064 3.52703 3.53288 3.5383 3.54248 3.54635 3.55067 3.55538 3.56162 3.56772 3.57355 3.57907 3.58466 3.59099 3.59795 3.60491 3.61176 3.61856 3.62438 3.62996 3.63625 3.64309 3.64978 3.65633 3.66344 3.67149 3.67995 3.68883 3.69977 3.7106 3.72128 3.72977 3.73862 3.74839 3.75854 3.76808 3.77731 3.78691 3.79724 3.80748 3.817 3.82465 3.83227 3.8402 3.84937 3.85948 3.87001 3.88001 3.88909 3.89708 3.90554 3.91623 3.9276 3.9408 3.95458 3.96671 3.97597 3.98588 3.99921 4.01279 4.02654 4.03959 4.05214 4.06294 4.07257 4.08033 4.08863 4.09953 4.11328 4.13091 4.15201 4.17387] V  V_range=[2.25 Inf] V  R0_mat=[0.75549 0.67245 0.17403 0.112;0.85269 0.75703 0.14702 0.03414;0.81792 0.71964 0.12022 0.00255;0.78315 0.68225 0.10415 2e-05;0.74837 0.64486 0.08835 2e-05;0.7136 0.60747 0.07462 2e-05;0.67883 0.57008 0.06392 2e-05;0.64406 0.53269 0.06243 0.01154;0.60929 0.49529 0.06276 0.02196;0.57452 0.4579 0.06157 0.02895;0.53975 0.42051 0.06015 0.03291;0.50498 0.38312 0.0587 0.03446;0.47021 0.34573 0.05791 0.03749;0.43544 0.30834 0.05742 0.03912;0.40067 0.27163 0.05726 0.04077;0.3659 0.2399 0.05695 0.04312;0.33113 0.21598 0.05669 0.04519;0.29855 0.19556 0.0563 0.04597;0.27187 0.18199 0.05643 0.04689;0.25149 0.16998 0.05637 0.04778;0.23672 0.15947 0.05613 0.04881;0.22094 0.15288 0.05627 0.04983;0.21055 0.14641 0.0562 0.05042;0.19955 0.13998 0.0555 0.04905;0.19137 0.13379 0.05463 0.04734;0.18464 0.13036 0.05424 0.0468;0.17901 0.12743 0.05396 0.04733;0.17336 0.12471 0.05353 0.04759;0.16963 0.12142 0.05325 0.04697;0.16579 0.11998 0.053 0.04616;0.16242 0.11856 0.05273 0.04563;0.15887 0.11696 0.05239 0.04515;0.15558 0.1153 0.05185 0.04523;0.15182 0.11319 0.05104 0.04515;0.14868 0.11098 0.05016 0.04495;0.14619 0.10898 0.0496 0.04427;0.1438 0.10712 0.04917 0.0435;0.14196 0.10583 0.049 0.0433;0.14006 0.10467 0.04873 0.04342;0.13885 0.1036 0.04841 0.04343;0.13751 0.10241 0.04805 0.04333;0.13605 0.10125 0.04775 0.04289;0.13479 0.10081 0.04765 0.04219;0.13386 0.10079 0.04766 0.04172;0.13314 0.10076 0.04767 0.04125;0.13237 0.10071 0.04767 0.04141;0.13163 0.10106 0.04767 0.04164;0.13057 0.10103 0.04746 0.04127;0.12942 0.10092 0.04718 0.04039;0.12835 0.0993 0.04683 0.03977;0.12742 0.09756 0.04661 0.03935;0.12651 0.09576 0.04638 0.03877;0.12576 0.09551 0.04611 0.03814;0.12522 0.09549 0.04546 0.03775;0.12534 0.0958 0.04498 0.03789;0.12567 0.09566 0.0446 0.03806;0.12544 0.09568 0.04436 0.03754;0.12563 0.09645 0.0447 0.03778;0.12579 0.09742 0.0452 0.03809;0.12561 0.09838 0.04568 0.03858;0.12463 0.09848 0.04568 0.03827;0.12444 0.09858 0.04565 0.03791;0.12488 0.09902 0.04553 0.03774;0.12541 0.0989 0.04551 0.03771;0.12553 0.09832 0.04545 0.0378;0.12554 0.09763 0.04533 0.03827;0.12569 0.09779 0.04532 0.03888;0.12679 0.09822 0.0455 0.03964;0.12813 0.09884 0.04565 0.03957;0.12921 0.09949 0.04568 0.03924;0.12875 0.09944 0.04547 0.03856;0.12761 0.09947 0.04525 0.03793;0.12678 0.09962 0.04509 0.0374;0.12741 0.10014 0.04486 0.03728;0.12819 0.10071 0.04471 0.03749;0.12866 0.10143 0.04473 0.03825;0.12934 0.10218 0.04488 0.0389;0.13071 0.10266 0.04509 0.03921;0.13167 0.10268 0.04508 0.03827;0.13235 0.10275 0.04519 0.03748;0.13367 0.10365 0.04567 0.03751;0.13524 0.10475 0.0459 0.03791;0.1378 0.10652 0.04653 0.03898;0.14098 0.10898 0.04736 0.0402;0.14355 0.11127 0.04774 0.04039;0.14492 0.11249 0.04743 0.03953;0.1465 0.11343 0.04723 0.03861;0.14934 0.11546 0.04771 0.03891;0.15255 0.11759 0.04823 0.0391;0.15585 0.12007 0.04878 0.03936;0.15888 0.12238 0.04933 0.0398;0.16256 0.12454 0.04973 0.04018;0.16629 0.12609 0.0497 0.03988;0.16958 0.1272 0.04945 0.03914;0.1737 0.12779 0.0488 0.0377;0.17938 0.12952 0.04782 0.03647;0.18591 0.1322 0.04663 0.0362;0.19342 0.13509 0.04586 0.03591;0.20235 0.13879 0.04557 0.03672;0.20886 0.14194 0.04146 0.03487;0.20094 0.13122 0.03511 0.0299] Ohm  R0_vec=[0.17403 0.14702 0.12022 0.10415 0.08835 0.07462 0.06392 0.06243 0.06276 0.06157 0.06015 0.0587 0.05791 0.05742 0.05726 0.05695 0.05669 0.0563 0.05643 0.05637 0.05613 0.05627 0.0562 0.0555 0.05463 0.05424 0.05396 0.05353 0.05325 0.053 0.05273 0.05239 0.05185 0.05104 0.05016 0.0496 0.04917 0.049 0.04873 0.04841 0.04805 0.04775 0.04765 0.04766 0.04767 0.04767 0.04767 0.04746 0.04718 0.04683 0.04661 0.04638 0.04611 0.04546 0.04498 0.0446 0.04436 0.0447 0.0452 0.04568 0.04568 0.04565 0.04553 0.04551 0.04545 0.04533 0.04532 0.0455 0.04565 0.04568 0.04547 0.04525 0.04509 0.04486 0.04471 0.04473 0.04488 0.04509 0.04508 0.04519 0.04567 0.0459 0.04653 0.04736 0.04774 0.04743 0.04723 0.04771 0.04823 0.04878 0.04933 0.04973 0.0497 0.04945 0.0488 0.04782 0.04663 0.04586 0.04557 0.04146 0.03511] Ohm  R0_dis_mat=[.0117, .0085, .009; .011, .0085, .009; .0114, .0087, .0092; .0107, .0082, .0088; .0107, .0083, .0091; .0113, .0085, .0089; .0116, .0085, .0089] % Parameter not set Ohm  R0_dis_vec=[.0085, .0085, .0087, .0082, .0083, .0085, .0085] % Parameter not set Ohm  R0_ch_mat=[.0117, .0085, .009; .011, .0085, .009; .0114, .0087, .0092; .0107, .0082, .0088; .0107, .0083, .0091; .0113, .0085, .0089; .0116, .0085, .0089] % Parameter not set Ohm  R0_ch_vec=[.0085, .0085, .0087, .0082, .0083, .0085, .0085] % Parameter not set Ohm  AH=260 hr*A  prm_leak=simscape.enum.tablebattery.prm_leak.disabled  Rleak_vec=[8000, 7000, 6000] % Parameter not set Ohm  Rleak=7e3 % Parameter not set Ohm  extrapolation_option=simscape.enum.extrapolation.nearest  SOC_port=simscape.enum.tablebattery.enable.no  prm_dyn=simscape.enum.tablebattery.prm_dyn.off  R1_mat=[.0109, .0029, .0013; .0069, .0024, .0012; .0047, .0026, .0013; .0034, .0016, .001; .0033, .0023, .0014; .0033, .0018, .0011; .0028, .0017, .0011] % Parameter not set Ohm  R1_vec=[.0029, .0024, .0026, .0016, .0023, .0018, .0017] % Parameter not set Ohm  tau1_mat=[20, 36, 39; 31, 45, 39; 109, 105, 61; 36, 29, 26; 59, 77, 67; 40, 33, 29; 25, 39, 33] % Parameter not set s  tau1_vec=[36, 45, 105, 29, 77, 33, 39] % Parameter not set s  R2_mat=[.0109, .0029, .0013; .0069, .0024, .0012; .0047, .0026, .0013; .0034, .0016, .001; .0033, .0023, .0014; .0033, .0018, .0011; .0028, .0017, .0011] % Parameter not set Ohm  R2_vec=[.0029, .0024, .0026, .0016, .0023, .0018, .0017] % Parameter not set Ohm  tau2_mat=[20, 36, 39; 31, 45, 39; 109, 105, 61; 36, 29, 26; 59, 77, 67; 40, 33, 29; 25, 39, 33] % Parameter not set s  tau2_vec=[36, 45, 105, 29, 77, 33, 39] % Parameter not set s  R3_mat=[.0109, .0029, .0013; .0069, .0024, .0012; .0047, .0026, .0013; .0034, .0016, .001; .0033, .0023, .0014; .0033, .0018, .0011; .0028, .0017, .0011] % Parameter not set Ohm  R3_vec=[.0029, .0024, .0026, .0016, .0023, .0018, .0017] % Parameter not set Ohm  tau3_mat=[20, 36, 39; 31, 45, 39; 109, 105, 61; 36, 29, 26; 59, 77, 67; 40, 33, 29; 25, 39, 33] % Parameter not set s  tau3_vec=[36, 45, 105, 29, 77, 33, 39] % Parameter not set s  R4_mat=[.0109, .0029, .0013; .0069, .0024, .0012; .0047, .0026, .0013; .0034, .0016, .001; .0033, .0023, .0014; .0033, .0018, .0011; .0028, .0017, .0011] % Parameter not set Ohm  R4_vec=[.0029, .0024, .0026, .0016, .0023, .0018, .0017] % Parameter not set Ohm  tau4_mat=[20, 36, 39; 31, 45, 39; 109, 105, 61; 36, 29, 26; 59, 77, 67; 40, 33, 29; 25, 39, 33] % Parameter not set s  tau4_vec=[36, 45, 105, 29, 77, 33, 39] % Parameter not set s  R5_mat=[.0109, .0029, .0013; .0069, .0024, .0012; .0047, .0026, .0013; .0034, .0016, .001; .0033, .0023, .0014; .0033, .0018, .0011; .0028, .0017, .0011] % Parameter not set Ohm  R5_vec=[.0029, .0024, .0026, .0016, .0023, .0018, .0017] % Parameter not set Ohm  tau5_mat=[20, 36, 39; 31, 45, 39; 109, 105, 61; 36, 29, 26; 59, 77, 67; 40, 33, 29; 25, 39, 33] % Parameter not set s  tau5_vec=[36, 45, 105, 29, 77, 33, 39] % Parameter not set s  prm_fade=simscape.enum.tablebattery.prm_fade.tableN  N0=100 % Parameter not set  dV0=0 % Parameter not set  dR0=0 % Parameter not set  dAH=0 % Parameter not set  dRleak=0 % Parameter not set  dR1=0 % Parameter not set  dR2=0 % Parameter not set  dR3=0 % Parameter not set  dR4=0 % Parameter not set  dR5=0 % Parameter not set  N0vec=[0 7 13 19 25 31 37 43 49 55 61 67 73 79 85 91 97 103 109 115 121 127 133 139 145 151 157 163 169 175 181 187 193 199 205 211 217 223 229 235 241 247 253 259 265 271 277 283 289 295 301 307 313 319 325 331 337 343 349 355 361 367 373 379 385 391 397 403 409 415 421 427 433 439 445 451 457 463 469 475 481 487 493 499]  Tfadevec=[298.15, 323.15] % Parameter not set K  dV0vec=[0 -0.2132 -0.4265 -0.6357 -0.8415 -1.0444 -1.2163 -1.3883 -1.52 -1.6273 -1.7347 -1.8294 -1.9144 -1.9994 -2.0744 -2.1392 -2.204 -2.2607 -2.3098 -2.3589 -2.408 -2.4643 -2.5252 -2.5861 -2.647 -2.7238 -2.8051 -2.8864 -2.9759 -3.0704 -3.1649 -3.261 -3.3591 -3.4573 -3.5079 -3.5566 -3.6065 -3.6564 -3.7063 -3.7562 -3.8061 -3.8559 -3.9166 -3.9805 -4.0444 -4.1083 -4.1723 -4.2352 -4.2979 -4.3605 -4.4214 -4.4739 -4.5206 -4.5597 -4.5988 -4.6379 -4.6769 -4.716 -4.7547 -4.7957 -4.8368 -4.8778 -4.9188 -4.9598 -5.0123 -5.066 -5.1196 -5.1598 -5.1853 -5.2109 -5.2365 -5.2631 -5.2922 -5.3213 -5.3503 -5.3816 -5.4144 -5.4471 -5.4798 -5.5126 -5.5453 -5.578 -5.6097 -5.641]  dR0vec=[0 0 0 0 0 0 0 0 0 0 0 0 0 0 0 0 0 0 0 0 0 0 0 0 0 0 0 0 0 0 0 0 0 0 0 0 0 0 0 0 0 0 0 0 0 0 0 0 0 0 0 0 0 0 0 0 0 0 0 0 0 0 0 0 0 0 0 0 0 0 0 0 0 0 0 0 0 0 0 0 0 0 0 0] % Parameter assumed  dAHvec=[0 -0.407 -0.814 -1.221 -1.629 -2.036 -2.443 -2.85 -3.207 -3.533 -3.859 -4.185 -4.51 -4.836 -5.162 -5.488 -5.813 -6.105 -6.369 -6.633 -6.897 -7.161 -7.425 -7.689 -7.953 -8.255 -8.569 -8.883 -9.197 -9.511 -9.826 -10.14 -10.454 -10.768 -10.93 -11.081 -11.233 -11.384 -11.536 -11.687 -11.838 -11.99 -12.176 -12.372 -12.569 -12.765 -12.962 -13.158 -13.354 -13.551 -13.741 -13.906 -14.07 -14.235 -14.399 -14.564 -14.728 -14.893 -15.06 -15.244 -15.429 -15.614 -15.799 -15.983 -16.168 -16.353 -16.538 -16.676 -16.764 -16.852 -16.94 -17.028 -17.116 -17.204 -17.292 -17.387 -17.486 -17.585 -17.684 -17.783 -17.883 -17.982 -18.081 -18.18]  dRleakvec=[0, 0, 0] % Parameter not set  dR1vec=[0, 0, 0] % Parameter not set  dR2vec=[0, 0, 0] % Parameter not set  dR3vec=[0, 0, 0] % Parameter not set  dR4vec=[0, 0, 0] % Parameter not set  dR5vec=[0, 0, 0] % Parameter not set  dV0mat=[0, 0; 0, 0; 0, 0] % Parameter not set  dR0mat=[0, 0; 0, 0; 0, 0] % Parameter not set  dAHmat=[0, 0; 0, 0; 0, 0] % Parameter not set  dRleakmat=[0, 0; 0, 0; 0, 0] % Parameter not set  dR1mat=[0, 0; 0, 0; 0, 0] % Parameter not set  dR2mat=[0, 0; 0, 0; 0, 0] % Parameter not set  dR3mat=[0, 0; 0, 0; 0, 0] % Parameter not set  dR4mat=[0, 0; 0, 0; 0, 0] % Parameter not set  dR5mat=[0, 0; 0, 0; 0, 0] % Parameter not set  prm_age_modeling=simscape.enum.tablebattery.prm_age_modeling.equation  storage_dt_age_vec=[0] % Parameter not set d  storage_T_age_vec=[273] % Parameter not set K  prm_age_OCV=simscape.enum.tablebattery.prm_age_OCV.OCV  OCV_age=0.9 % Parameter not set  SOC_age=0.6 % Parameter not set  prm_age_resistance=simscape.enum.tablebattery.prm_age.disabled  OCV_scaling_age_resistance=2.2134e6 % Parameter not set  OCV_offset_age_resistance=1.632e6 % Parameter not set  temp_exp_age_resistance=0.515833569 % Parameter not set V  t_exp_age_resistance=0.75 % Parameter not set  T_age_vec_resistance=[273.15, 298.15, 323.15] % Parameter not set K  dt_age_vec_resistance=[90, 180, 270, 360] % Parameter not set d  dR0_age_vec=[0, 0, 0] % Parameter not set  t_meas_dR0_age=100 % Parameter not set d  dR0_age_mat=[0, 0, 0; 0, 0, 0; 0, 0, 0; 0, 0, 0] % Parameter not set  prm_age_capacity=simscape.enum.tablebattery.prm_age.disabled  OCV_scaling_age_capacity=1.5097e07 % Parameter not set  OCV_offset_age_capacity=8.3625e06 % Parameter not set  temp_exp_age_capacity=0.6011 % Parameter not set V  t_exp_age_capacity=0.75 % Parameter not set  T_age_vec_capacity=[273.15, 298.15, 323.15] % Parameter not set K  dt_age_vec_capacity=[90, 180, 270, 360] % Parameter not set d  dAH_age_vec=[0, 0, 0] % Parameter not set  t_meas_dAH_age=100 % Parameter not set d  dAH_age_mat=[0, 0, 0; 0, 0, 0; 0, 0, 0; 0, 0, 0] % Parameter not set  thermal_port=simscape.enum.thermaleffects.model  temperature=298.15 % Parameter not set K  thermal_mass=43.2 % Parameter assumed J/K  i_specify=off  i_priority=None  i=0 A  i_nominal_specify=off  i_nominal_unit=A  i_nominal_value=1  v_specify=off  v_priority=None  v=0 V  v_nominal_specify=off  v_nominal_unit=V  v_nominal_value=1  stateOfCharge_specify=off  stateOfCharge_priority=High  stateOfCharge=1  stateOfCharge_nominal_specify=off  stateOfCharge_nominal_unit=1  stateOfCharge_nominal_value=1  num_cycles_specify=off  num_cycles_priority=High  num_cycles=0  num_cycles_nominal_specify=off  num_cycles_nominal_unit=1  num_cycles_nominal_value=1  cell_temperature_specify=off  cell_temperature_priority=High  cell_temperature=298.15 K  cell_temperature_nominal_specify=off  cell_temperature_nominal_unit=K  cell_temperature_nominal_value=1
      settings: AttributesFormatString=Panasonic:NCR18650PF  InternalSimscapePortConfiguration="{\"Bottom\":[],\"Left\":[{\"id\":\"p\",\"label\":\"+\",\"type\":\"foundation.electrical.electrical\"}],\"Right\":[{\"id\":\"n\",\"label\":\"-\",\"type\":\"foundation.electrical.electrical\"},{\"id\":\"H\",\"label\":\"H\",\"type\":\"foundation.thermal.thermal\"}],\"Top\":[]}"
      settings: LibrarySourceBlock=|
      | batt_lib/Cells/Battery
      | (Table-Based)
  PS-Simulink Converter : nesl_utility/PS-Simulink Converter  PhysicalDomain=network_engine_domain  SubClassName=ps_output  LeftPortType=input  RightPortType=output  PseudoPeriodic=off  Frequencies=[]  VectorFormat=inherit  Unit=inherit  AffineConversion=off
  + : PMIOPort  Side=Left
  - : PMIOPort  Port=2  Side=Right
  SOC : Outport
  wires:
  PS-Simulink Converter/1 -> SOC/1
  connections:
  Battery (Table-Based)3/LConn1 -- Battery (Table-Based)2/RConn1
  Battery (Table-Based)1/LConn1 -- Battery (Table-Based)/RConn1
  Battery (Table-Based)2/LConn1 -- Battery (Table-Based)1/RConn1
  Battery (Table-Based)/LConn1 -- +/RConn1
  Battery (Table-Based)5/LConn1 -- Battery (Table-Based)4/RConn1
  Battery (Table-Based)4/LConn1 -- Battery (Table-Based)3/RConn1
  Battery (Table-Based)7/LConn1 -- Battery (Table-Based)6/RConn1
  Battery (Table-Based)6/LConn1 -- Battery (Table-Based)5/RConn1
  Battery (Table-Based)9/LConn1 -- Battery (Table-Based)8/RConn1
  Battery (Table-Based)8/LConn1 -- Battery (Table-Based)7/RConn1
  Battery (Table-Based)9/RConn1 -- Battery (Table-Based)11/LConn1
  Battery (Table-Based)13/LConn1 -- Battery (Table-Based)12/RConn1
  Battery (Table-Based)12/LConn1 -- Battery (Table-Based)11/RConn1
  -/RConn1 -- Battery (Table-Based)17/RConn1
  Battery (Table-Based)25/LConn1 -- Battery (Table-Based)24/RConn1
  Battery (Table-Based)22/LConn1 -- Battery (Table-Based)21/RConn1
  Battery (Table-Based)24/LConn1 -- Battery (Table-Based)23/RConn1
  Battery (Table-Based)17/LConn1 -- Battery (Table-Based)16/RConn1
  Battery (Table-Based)27/LConn1 -- Battery (Table-Based)26/RConn1
  Battery (Table-Based)21/LConn1 -- Battery (Table-Based)20/RConn1
  Battery (Table-Based)15/LConn1 -- Battery (Table-Based)14/RConn1
  Battery (Table-Based)26/LConn1 -- Battery (Table-Based)25/RConn1
  Battery (Table-Based)20/LConn1 -- Battery (Table-Based)15/RConn1
  Battery (Table-Based)23/LConn1 -- Battery (Table-Based)22/RConn1
  Battery (Table-Based)16/LConn1 -- Battery (Table-Based)27/RConn1
  Battery (Table-Based)14/LConn1 -- Battery (Table-Based)13/RConn1
  Battery (Table-Based)/LConn2 -- PS-Simulink Converter/LConn1
